simulink model "test_1"  (R2014a)
settings: Solver=ode45  StartTime=0.0  StopTime=100  RelTol=1e-3
libraries: simulink x1
settings Model: Creator=BIgC46263347  LastModifiedBy=BIgC46263347

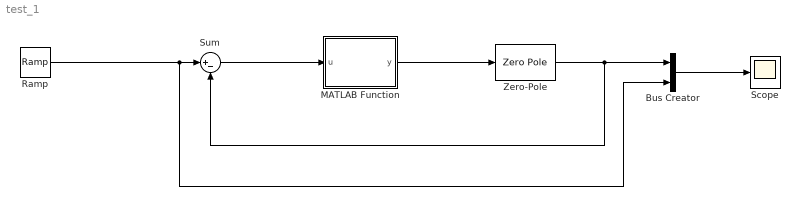
== system test_1 ==
  Bus Creator : BusCreator  Inputs=2
  MATLAB Function : MATLAB Function  TreatAsAtomicUnit=on
  Ramp : simulink/Sources/Ramp  slope=1  start=0  X0=0
  Scope : Scope
  Sum : Sum  Inputs=|+-
  Zero-Pole : ZeroPole  Zeros=[]  Poles=[-1/20]  Gain=[1/10]
  wires:
  MATLAB Function/1(y) -> Zero-Pole/1
  Bus Creator/1 -> Scope/1
  Sum/1 -> MATLAB Function/1(u)
  Zero-Pole/1 -> Sum/2, Bus Creator/1
  Ramp/1 -> Bus Creator/2, Sum/1

== matlab function test_1/MATLAB Function ==
  data: u input; y output
function y = fcn(u)
gap=0.5;

y=u;
if (u>gap)
    y=u;
elseif(u<-gap)
    y=0;
end
    
    

end
